simulink model "q3w3"  (R2024b)
settings: Solver=VariableStepAuto  StartTime=0.0  StopTime=10.0  RelTol=1e-3

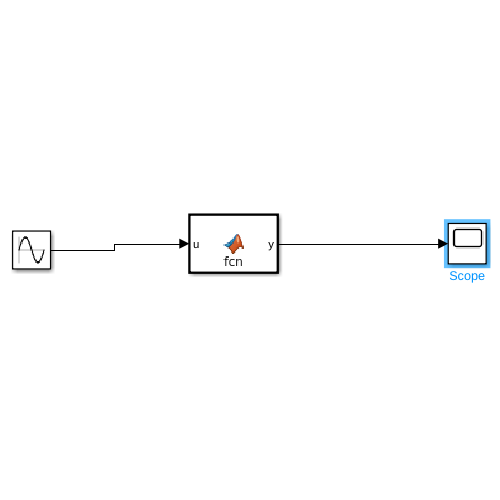
[thumbnail: Simulink's stored preview of the top-level diagram]
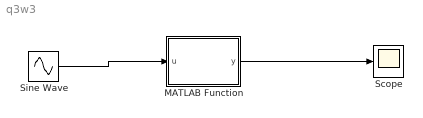
== system q3w3 ==
  MATLAB Function : MATLAB Function  TreatAsAtomicUnit=on
  Scope : Scope
  Sine Wave : Sin  Frequency=6.28  SampleTime=0
  wires:
  Sine Wave/1 -> MATLAB Function/1(u)
  MATLAB Function/1(y) -> Scope/1

== matlab function q3w3/MATLAB Function ==
  data: u input; y output
function y = fcn(u)

y = 2*u^2+3*sin(u)-5;
